simulink model "BugE_v0_40_MAS"  (R2015b)
settings: Solver=FixedStepDiscrete  StartTime=0.0  StopTime=inf  FixedStep=sample_time  RelTol=1e-3
values from neighbouring files (symbols this model uses):
  AB_diode_dV = 0.9    [main_sync.m]
  air_density = 1.225    [main_sync.m]
  bus_charger_Pmax = 1000    [main_sync.m]
  bus_load_Pmax_abs = 500    [main_sync.m]
  capInitVolt = capVmax*sqrt(capInitSoC)    [main_sync.m]
  cyc_kph = [cyc_kph(:,1), cyc_kph(:,2)*speed_max_limit/speed_max]    [main_sync.m]
  cyc_repeat = 0    [main_sync.m]
  ess1_init_soc = 1    [main_sync.m]
  ess1_soh = 1    [main_sync.m]
  ess2_init_soc = 1    [main_sync.m]
  ess2_soh = 1    [main_sync.m]
  ess3_init_soc = 1    [main_sync.m]
  ess3_soh = 1    [main_sync.m]
  ess4_init_soc = 1    [main_sync.m]
  ess4_soh = 1    [main_sync.m]
  ess5_init_soc = 1    [main_sync.m]
  ess5_soh = 1    [main_sync.m]
  gear_ratio = 6    [main_sync.m]
  loadpower = rawcsv(:,2)    [main_sync.m]
  loadtime = rawcsv(:,1)    [main_sync.m]
  lockSOCs = 0    [main_sync.m]
  max_brk_torque = 300    [main_sync.m]
  no_wheels = 3    [main_sync.m]
  period2 = max(loadtime)    [main_sync.m]
  PV_Pmax = 100    [main_sync.m]
  sample_time = 0.01    [main_sync.m]
  startup_seq_step_delay = 0.2    [main_sync.m]
  stop_option = 0    [main_sync.m]
  use_drive_cycle = 1    [main_sync.m]
  use_real_subs_loads = 1    [main_sync.m]
  vbus_max = 25    [main_sync.m]
  vbus_min = 17    [main_sync.m]
  vbus_safety_threshold = 2    [main_sync.m]
  vbus_threshold = 20    [main_sync.m]
  veh_CD = 0.35    [main_sync.m]
  veh_FA = 1.543    [main_sync.m]
  veh_gravity = 9.81*veh_mass    (= 1863.9)    [main_sync.m]
  veh_mass = 190    [main_sync.m]
  wh_1st_rrc = 0.02    [main_sync.m]
  wh_bearing_frc = 0.0015    [main_sync.m]
  wh_inertia = 0.0556    [main_sync.m]
  wh_radius = 0.508/2    (= 0.254)    [main_sync.m]
undefined symbols (not defined in the file or in its folder): capC, capR, cyc_acc, cyc_avg_time_samples, cyc_brk, cyc_grade, cyc_key, DCM_eff_factor_for_Vin, DCM_eff_for_Iout, DCM_Iout, DCM_Iout_max, DCM_Pin_noload, DCM_Pout_max, DCM_Vin, DCM_Vout, DiscIntNeverNeededParam, ess2_coulombic_eff, ess2_Ineg_max_SOC, ess2_Ineg_max_temp, ess2_Ipos_max_SOC, ess2_Ipos_max_temp, ess2_max_ah_cap, ess2_max_volts, ess2_min_volts, ess2_module_parallel, ess2_module_series, ess2_r_dis, ess2_soc, ess2_SOC_for_Ilimit, ess2_temp_for_Ilimit, ess2_temp_max, ess2_tmp, ess2_voc, ess3_coulombic_eff, ess3_max_ah_cap, ess3_module_parallel, ess3_module_series, ess3_r_dis, ess3_soc, ess3_tmp, ess3_voc, ess_coulombic_eff, ess_Ineg_max_SOC, ess_Ineg_max_temp, ess_Ipos_max_SOC, ess_Ipos_max_temp, ess_max_ah_cap, ess_max_volts, ess_min_volts, ess_module_parallel, ess_module_series, ess_nominal_volts, ess_r_dis, ess_soc, ess_SOC_for_Ilimit, ess_temp_for_Ilimit, ess_temp_max, ess_tmp, ess_voc, MC_eff1 ... (+17)
libraries: simulink x139, commfilt2 x1, simulink_extras x1
(part 6 of 7)

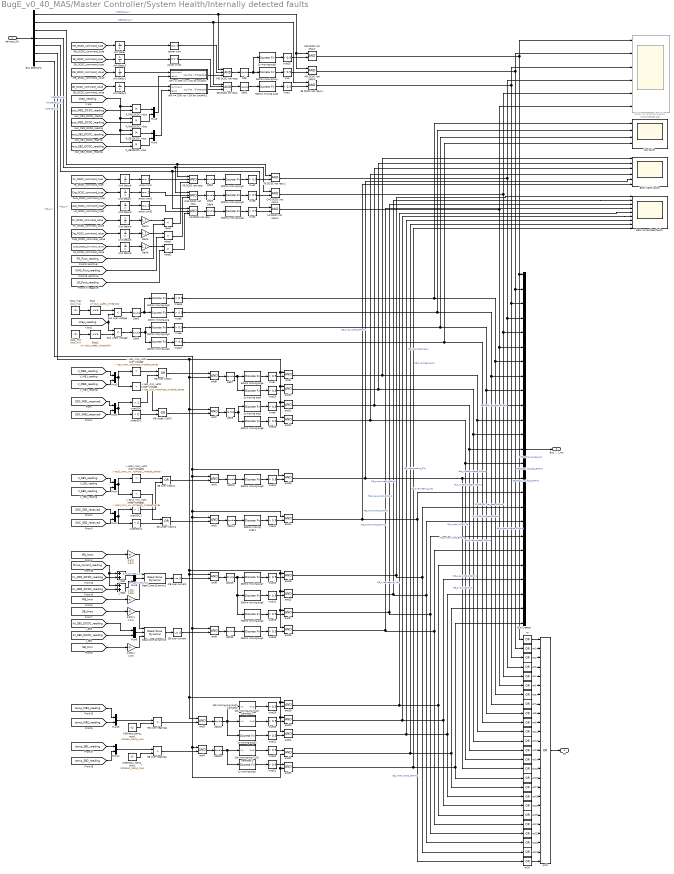
== system BugE_v0_40_MAS/Master Controller/System Health/Internally detected faults ==
  devices_ON : Inport
  0.90*ess2_temp_max1 : Constant  Value=0.9*ess2_temp_max  SampleTime=sample_time
  0.90*ess_temp_max1 : Constant  Value=0.9*ess_temp_max  SampleTime=sample_time
  "0.975 " : Gain  Gain=0.975
  0.975 1 : Gain  Gain=0.975
  "1.025 " : Gain  Gain=1.025
  1.025 1 : Gain  Gain=1.025
  1s moving avg{1..4,20} (5 alike) : DiscreteFir  Coefficients=ones(1,1*(1/sample_time))/(1*(1/sample_time))  SampleTime=sample_time
  200ms moving avg : DiscreteFir  Coefficients=ones(1,0.2*(1/sample_time))/(0.2*(1/sample_time))  SampleTime=sample_time
  200ms moving avg1 : DiscreteFir  Coefficients=ones(1,0.2*(1/sample_time))/(0.2*(1/sample_time))  SampleTime=sample_time
  20s moving avg (1/20 samples)1 : Subsystem
  20s moving avg (1/20 samples)3 : Subsystem
  250ms moving avg1 : DiscreteFir  Coefficients=ones(1,0.25*(1/sample_time))/(0.25*(1/sample_time))  SampleTime=sample_time
  250ms moving avg7 : DiscreteFir  Coefficients=ones(1,0.25*(1/sample_time))/(0.25*(1/sample_time))  SampleTime=sample_time
  2dbl{,1..7,9,12,14..16,19..20} (15 alike) : DataTypeConversion  OutDataTypeStr=double
  400ms moving avg1 : DiscreteFir  Coefficients=ones(1,0.4*(1/sample_time))/(0.4*(1/sample_time))  SampleTime=sample_time
  400ms moving avg2 : DiscreteFir  Coefficients=ones(1,0.4*(1/sample_time))/(0.4*(1/sample_time))  SampleTime=sample_time
  40s moving avg (1/40 samples) : Subsystem
  500ms moving avg{,1..6,8..9,11} (10 alike) : DiscreteFir  Coefficients=ones(1,0.5*(1/sample_time))/(0.5*(1/sample_time))  SampleTime=sample_time
  750ms moving avg2 : DiscreteFir  Coefficients=ones(1,0.75*(1/sample_time))/(0.75*(1/sample_time))  SampleTime=sample_time
  < ess2_min_volts under-voltage1 : simulink/Logic and Bit Operations/Compare To Constant  relop=<  const=ess2_min_volts*ess2_module_series  OutDataTypeStr=boolean
  < ess_min_volts under-voltage : simulink/Logic and Bit Operations/Compare To Constant  relop=<  const=ess_min_volts*ess_module_series  OutDataTypeStr=boolean
  > ess2_max_volts over-voltage1 : simulink/Logic and Bit Operations/Compare To Constant  relop=>  const=ess2_max_volts*ess2_module_series  OutDataTypeStr=boolean
  > ess_max_volts over-voltage : simulink/Logic and Bit Operations/Compare To Constant  relop=>  const=ess_max_volts*ess_module_series  OutDataTypeStr=boolean
  Batt V/SOC faults : Scope  NumInputPorts=6
  Batt current/heat faults : Scope  NumInputPorts=9
  Bias : Bias  Bias=vbus_safety_threshold
  Bias1 : Bias  Bias=-vbus_safety_threshold
  Bus Creator : BusCreator  Inputs=25
  Bus Selector3 : BusSelector  OutputSignals=MBDCDC_on,SBDCDC_on,FEDCDC_on,CHGDCDC_on,LDDCDC_on,MB_on,SB_on
  Bus over voltage : RelationalOperator  Operator=<  OutDataTypeStr=boolean
  Bus under voltage : RelationalOperator  Operator=<  OutDataTypeStr=boolean
  CHG DCDC not resp. : Logic  Inputs=3  AllPortsSameDT=off  OutDataTypeStr=boolean
  CHG DCDC not resp.1 : Logic  AllPortsSameDT=off  OutDataTypeStr=boolean
  DCDC not responding faults : Scope  Commented=on  NumInputPorts=6
  Dead Zone Dynamic2 : simulink/Discontinuities/Dead Zone Dynamic
  Dead Zone Dynamic3 : simulink/Discontinuities/Dead Zone Dynamic
  FE DCDC not resp. : Logic  Inputs=3  AllPortsSameDT=off  OutDataTypeStr=boolean
  FE DCDC not resp.1 : Logic  AllPortsSameDT=off  OutDataTypeStr=boolean
  Gain4 : Gain  Gain=1.1
  Gain5 : Gain  Gain=1.1
  Gain6 : Gain  Gain=1.1
  I_MB1 : Sum
  I_MB2 : Sum
  LD DCDC not resp. : Logic  Inputs=3  AllPortsSameDT=off  OutDataTypeStr=boolean
  LD DCDC not resp.1 : Logic  AllPortsSameDT=off  OutDataTypeStr=boolean
  MB over-heating1 : RelationalOperator  Operator=>  OutDataTypeStr=boolean
  MB DCDC not resp. : Logic  Inputs=3  AllPortsSameDT=off  OutDataTypeStr=boolean
  MB DCDC not resp.1 : Logic  AllPortsSameDT=off  OutDataTypeStr=boolean
  MB DCDC not resp.2 : Logic  AllPortsSameDT=off  OutDataTypeStr=boolean
  MB over V/SOC : Logic  Operator=OR  AllPortsSameDT=off  OutDataTypeStr=boolean
  MB over-current : simulink/Logic and Bit Operations/Compare To Zero  relop=~=  OutDataTypeStr=boolean
  MB under V/SOC : Logic  Operator=OR  AllPortsSameDT=off  OutDataTypeStr=boolean
  Mux{1..6,8..9,13..14} (10 alike) : Mux  Inputs=2
  P_MB1DCDC->bus : Product
  P_MB2DCDC->bus : Product
  P_SB1DCDC->bus : Product
  P_SB2DCDC->bus : Product
  SB over-heating1 : RelationalOperator  Operator=>  OutDataTypeStr=boolean
  SB DCDC not resp. : Logic  Inputs=3  AllPortsSameDT=off  OutDataTypeStr=boolean
  SB DCDC not resp.1 : Logic  AllPortsSameDT=off  OutDataTypeStr=boolean
  SB over V/SOC1 : Logic  Operator=OR  AllPortsSameDT=off  OutDataTypeStr=boolean
  SB over-current : simulink/Logic and Bit Operations/Compare To Zero  relop=~=  OutDataTypeStr=boolean
  SB under V/SOC1 : Logic  Operator=OR  AllPortsSameDT=off  OutDataTypeStr=boolean
  Unit Delay{,1..9} (10 alike) : UnitDelay  SampleTime=sample_time
  and{1..23} (23 alike) : Logic  AllPortsSameDT=off  OutDataTypeStr=boolean
  bus faults : Scope  NumInputPorts=4
  diff >= 10% (or >1W for cmd=0) : Subsystem
  diff >= 10% (or >1W for cmd=0)1 : Subsystem
  or{,1..9,11..25} (25 alike) : Logic  Operator=OR  Inputs=1  AllPortsSameDT=off  OutDataTypeStr=boolean
  or10 : Logic  Operator=OR  Inputs=25  AllPortsSameDT=off  OutDataTypeStr=boolean
  overSOC : simulink/Logic and Bit Operations/Compare To Constant  relop=>  const=1  OutDataTypeStr=boolean
  overSOC1 : simulink/Logic and Bit Operations/Compare To Constant  relop=>  const=1  OutDataTypeStr=boolean
  pmax cmd : simulink/Logic and Bit Operations/Compare To Constant  relop===  const=2  OutDataTypeStr=boolean
  pmax cmd1 : simulink/Logic and Bit Operations/Compare To Constant  relop===  const=2  OutDataTypeStr=boolean
  pmax cmd2 : simulink/Logic and Bit Operations/Compare To Constant  relop===  const=2  OutDataTypeStr=boolean
  power cmd : simulink/Logic and Bit Operations/Compare To Constant  relop===  const=0  OutDataTypeStr=boolean
  power cmd1 : simulink/Logic and Bit Operations/Compare To Constant  relop===  const=0  OutDataTypeStr=boolean
  relop : RelationalOperator  Operator=<  OutDataTypeStr=boolean
  relop1 : RelationalOperator  Operator=<  OutDataTypeStr=boolean
  relop2 : RelationalOperator  Operator=>  OutDataTypeStr=boolean
  true{,1..7,9..16,19..23,25..27,29} (25 alike) : simulink/Logic and Bit Operations/Compare To Constant  relop=>  const=0.5  OutDataTypeStr=boolean
  underSOC : simulink/Logic and Bit Operations/Compare To Constant  relop=<  const=0  OutDataTypeStr=boolean
  underSOC1 : simulink/Logic and Bit Operations/Compare To Constant  relop=<  const=0  OutDataTypeStr=boolean
  vbus_max : Constant  Value=vbus_max  SampleTime=sample_time
  vbus_min : Constant  Value=vbus_min  SampleTime=sample_time
  FD : Outport  SampleTime=sample_time
  Bus (...)_ms : Outport  Port=2  SampleTime=sample_time
  wires:
  diff >= 10% (or >1W for cmd=0)1/1(significant diff detected) -> SB DCDC not resp./3
  power cmd1/1 -> SB DCDC not resp./2
  Mux8/1 -> diff >= 10% (or >1W for cmd=0)/2(result)
  Mux9/1 -> diff >= 10% (or >1W for cmd=0)1/2(result)
  power cmd/1 -> MB DCDC not resp./2
  [MB_DCDC_command_type] -> Unit Delay/1
  [MB_DCDC_command_value] -> Unit Delay1/1
  [SB_DCDC_command_value] -> Unit Delay2/1
  [SB_DCDC_command_type] -> Unit Delay3/1
  [Iout_MB1_DCDC_reading] -> P_MB1DCDC->bus/2
  [Vcap_reading] -> P_MB1DCDC->bus/1, P_MB2DCDC->bus/1, P_SB1DCDC->bus/1, P_SB2DCDC->bus/1
  [Iout_MB2_DCDC_reading] -> P_MB2DCDC->bus/2
  [Iout_SB1_DCDC_reading] -> P_SB1DCDC->bus/2
  [Iout_SB2_DCDC_reading] -> P_SB2DCDC->bus/2
  Unit Delay/1 -> power cmd/1
  Unit Delay3/1 -> power cmd1/1
  P_MB1DCDC->bus/1 -> Mux8/1
  P_MB2DCDC->bus/1 -> Mux8/2
  P_SB1DCDC->bus/1 -> Mux9/1
  P_SB2DCDC->bus/1 -> Mux9/2
  Unit Delay1/1 -> diff >= 10% (or >1W for cmd=0)/1(command)
  Unit Delay2/1 -> diff >= 10% (or >1W for cmd=0)1/1(command)
  SB DCDC not resp./1 -> 2dbl1/1
  MB DCDC not resp./1 -> 2dbl/1
  vbus_min/1 -> Bias1/1
  vbus_max/1 -> Bias/1
  Bias/1 -> Bus over voltage/1
  [Vcap_reading] -> Bus over voltage/2, Bus under voltage/1
  Bias1/1 -> Bus under voltage/2
  [V_MB1_reading] -> Mux3/1
  [V_MB2_reading] -> Mux3/2
  [V_SB1_reading] -> Mux4/1
  [V_SB2_reading] -> Mux4/2
  [SOC_MB1_received] -> Mux1/1
  [SOC_MB2_received] -> Mux1/2
  Mux1/1 -> overSOC/1, underSOC/1
  Mux3/1 -> > ess_max_volts over-voltage/1, < ess_min_volts under-voltage/1
  > ess_max_volts over-voltage/1 -> MB over V/SOC/1
  overSOC/1 -> MB over V/SOC/2
  underSOC/1 -> MB under V/SOC/2
  < ess_min_volts under-voltage/1 -> MB under V/SOC/1
  [SOC_SB2_received] -> Mux2/2
  [SOC_SB1_received] -> Mux2/1
  and7/1 -> 2dbl9/1
  Mux5/1 -> Dead Zone Dynamic2/2
  [Iin_SB1_DCDC_reading] -> Mux6/1
  [Iin_SB2_DCDC_reading] -> Mux6/2
  Mux6/1 -> Dead Zone Dynamic3/2
  "0.975 "/1 -> Dead Zone Dynamic2/1
  "1.025 "/1 -> Dead Zone Dynamic2/3
  0.975 1/1 -> Dead Zone Dynamic3/1
  [MB_Imin] -> "1.025 "/1
  [MB_Imax] -> "0.975 "/1
  Dead Zone Dynamic3/1 -> SB over-current/1
  [Drive_current_reading] -> I_MB2/1, I_MB1/1
  [SB_Imax] -> 0.975 1/1
  [SB_Imin] -> 1.025 1/1
  1.025 1/1 -> Dead Zone Dynamic3/3
  I_MB1/1 -> Mux5/1  "ems_SH_MB1_Iout"
  [Iin_MB2_DCDC_reading] -> I_MB2/2
  [Iin_MB1_DCDC_reading] -> I_MB1/2
  I_MB2/1 -> Mux5/2  "ems_SH_MB2_Iout"
  [PV_DCDC_command_value] -> Unit Delay4/1
  [Chg_DCDC_command_value] -> Unit Delay5/1
  [PV_DCDC_command_type] -> Unit Delay6/1
  [Chg_DCDC_command_type] -> Unit Delay7/1
  [Load_DCDC_command_value] -> Unit Delay8/1
  [Load_DCDC_command_type] -> Unit Delay9/1
  Unit Delay6/1 -> pmax cmd/1
  Unit Delay7/1 -> pmax cmd1/1
  Unit Delay9/1 -> pmax cmd2/1
  Unit Delay4/1 -> Gain4/1
  Unit Delay5/1 -> Gain5/1
  Unit Delay8/1 -> Gain6/1
  Gain4/1 -> relop/1
  [FE_Pout_reading] -> relop/2
  Gain5/1 -> relop1/1
  [CHG_Pout_reading] -> relop1/2
  Gain6/1 -> relop2/1
  [LD_Pout_reading] -> relop2/2
  pmax cmd/1 -> FE DCDC not resp./2
  relop/1 -> FE DCDC not resp./3
  pmax cmd1/1 -> CHG DCDC not resp./2
  relop1/1 -> CHG DCDC not resp./3
  pmax cmd2/1 -> LD DCDC not resp./2
  relop2/1 -> LD DCDC not resp./3
  FE DCDC not resp./1 -> 2dbl2/1
  CHG DCDC not resp./1 -> 2dbl3/1
  LD DCDC not resp./1 -> 2dbl4/1
  500ms moving avg/1 -> true/1
  2dbl/1 -> 1s moving avg3/1, 500ms moving avg/1
  500ms moving avg1/1 -> true1/1
  2dbl1/1 -> 500ms moving avg1/1
  500ms moving avg2/1 -> true2/1
  2dbl2/1 -> 500ms moving avg2/1
  500ms moving avg3/1 -> true3/1
  2dbl3/1 -> 500ms moving avg3/1
  500ms moving avg4/1 -> true4/1
  2dbl4/1 -> 500ms moving avg4/1
  MB DCDC not resp.1/1 -> or1/1, Bus Creator/2, DCDC not responding faults/2  "MBDCDC_not_resp_500ms"
  FE DCDC not resp.1/1 -> or3/1, Bus Creator/4, DCDC not responding faults/4  "FEDCDC_not_resp_500ms"
  CHG DCDC not resp.1/1 -> or4/1, Bus Creator/5, DCDC not responding faults/5  "CHGDCDC_not_resp_500ms"
  LD DCDC not resp.1/1 -> or5/1, Bus Creator/6, DCDC not responding faults/6  "LD_DCDC_not_resp_500ms"
  200ms moving avg/1 -> true5/1
  2dbl5/1 -> 400ms moving avg2/1, 200ms moving avg/1
  true5/1 -> bus faults/2, or7/1, Bus Creator/8  "Bus_over-voltage_200ms"
  200ms moving avg1/1 -> true6/1
  2dbl6/1 -> 200ms moving avg1/1, 400ms moving avg1/1
  true6/1 -> bus faults/3, or8/1, Bus Creator/9  "Bus_under-voltage_200ms"
  500ms moving avg5/1 -> true7/1
  2dbl7/1 -> 1s moving avg4/1, 500ms moving avg5/1
  and5/1 -> Batt V/SOC faults/1, or11/1, Bus Creator/11  "MB_over_V/SOC_500ms"
  and10/1 -> Batt V/SOC faults/2, or12/1, Bus Creator/12  "MB_over_V/SOC_1s"
  1s moving avg2/1 -> true9/1
  and11/1 -> Batt V/SOC faults/3, or13/1, Bus Creator/13  "MB_under_V/SOC_1s"
  and12/1 -> Batt V/SOC faults/4, or14/1, Bus Creator/14  "MB_under_V/SOC_500ms"
  Mux2/1 -> overSOC1/1, underSOC1/1
  Mux4/1 -> > ess2_max_volts over-voltage1/1, < ess2_min_volts under-voltage1/1
  underSOC1/1 -> SB under V/SOC1/2
  < ess2_min_volts under-voltage1/1 -> SB under V/SOC1/1
  SB under V/SOC1/1 -> and2/2
  500ms moving avg9/1 -> true12/1
  2dbl12/1 -> 500ms moving avg9/1
  and13/1 -> Batt V/SOC faults/5, or15/1, Bus Creator/15  "SB_over_V/SOC_500ms"
  500ms moving avg11/1 -> true14/1
  2dbl14/1 -> 500ms moving avg11/1
  and14/1 -> Batt V/SOC faults/6, Bus Creator/16, or25/1  "SB_under_V/SOC_500ms"
  250ms moving avg7/1 -> true15/1
  2dbl15/1 -> 250ms moving avg7/1, 750ms moving avg2/1, 500ms moving avg6/1
  and8/1 -> 2dbl15/1
  and18/1 -> Batt current/heat faults/1, or24/1, Bus Creator/17  "MB_over-current_250ms"
  250ms moving avg1/1 -> true16/1
  2dbl16/1 -> 250ms moving avg1/1
  and9/1 -> 2dbl16/1
  and16/1 -> or21/1, Bus Creator/20, Batt current/heat faults/4  "SB_over-current_250ms"
  and21/1 -> or18/1, Bus Creator/23, Batt current/heat faults/7  "MB_over-heating_1s"
  and23/1 -> Batt current/heat faults/9, Bus Creator/25, or16/1  "SB_over-heating_1s"
  and20/1 -> or19/1, Bus Creator/22, Batt current/heat faults/6  "MB_over-heating_20s"
  and22/1 -> Batt current/heat faults/8, Bus Creator/24, or17/1  "SB_over-heating_20s"
  or10/1 -> FD/1
  or/1 -> or10/1
  or1/1 -> or10/2
  or2/1 -> or10/3
  or3/1 -> or10/4
  or4/1 -> or10/5
  or5/1 -> or10/6
  or6/1 -> or10/7
  or7/1 -> or10/8
  or8/1 -> or10/9
  or9/1 -> or10/10
  or11/1 -> or10/11
  or12/1 -> or10/12
  or13/1 -> or10/13
  or14/1 -> or10/14
  or15/1 -> or10/15
  or16/1 -> or10/16
  or17/1 -> or10/17
  or18/1 -> or10/18
  or19/1 -> or10/19
  or20/1 -> or10/20
  or21/1 -> or10/21
  true26/1 -> bus faults/1, or6/1, Bus Creator/7  "Bus_over-voltage_400ms"
  true27/1 -> bus faults/4, or9/1, Bus Creator/10  "Bus_under-voltage_400ms"
  Bus Creator/1 -> Bus (...)_ms/1
  1s moving avg4/1 -> true23/1
  500ms moving avg8/1 -> true10/1
  2dbl9/1 -> 1s moving avg2/1, 500ms moving avg8/1
  and15/1 -> Batt current/heat faults/2, or23/1, Bus Creator/18  "MB_over-current_500ms"
  500ms moving avg6/1 -> true11/1
  750ms moving avg2/1 -> true13/1
  and17/1 -> or22/1, Bus Creator/19, Batt current/heat faults/3  "MB_over-current_750ms"
  1s moving avg3/1 -> true25/1
  400ms moving avg2/1 -> true26/1
  400ms moving avg1/1 -> true27/1
  and19/1 -> Batt current/heat faults/5, or20/1, Bus Creator/21  "MB_over-heating_40s"
  or22/1 -> or10/22
  or23/1 -> or10/23
  or24/1 -> or10/24
  or25/1 -> or10/25
  > ess2_max_volts over-voltage1/1 -> SB over V/SOC1/1
  overSOC1/1 -> SB over V/SOC1/2
  diff >= 10% (or >1W for cmd=0)/1(significant diff detected) -> MB DCDC not resp./3
  Bus under voltage/1 -> 2dbl6/1
  Bus over voltage/1 -> 2dbl5/1
  SB over V/SOC1/1 -> and1/2
  devices_ON/1 -> Bus Selector3/1
  Bus Selector3/1 -> MB DCDC not resp.1/1, MB DCDC not resp.2/1, MB DCDC not resp./1  "<MBDCDC_on>"
  Bus Selector3/2 -> SB DCDC not resp.1/1, SB DCDC not resp./1  "<SBDCDC_on>"
  Bus Selector3/3 -> FE DCDC not resp.1/1, FE DCDC not resp./1  "<FEDCDC_on>"
  Bus Selector3/4 -> CHG DCDC not resp.1/1, CHG DCDC not resp./1  "<CHGDCDC_on>"
  Bus Selector3/5 -> LD DCDC not resp.1/1, LD DCDC not resp./1  "<LDDCDC_on>"
  Bus Selector3/6 -> and12/1, and11/1, and10/1, and5/1, and6/2, and7/1, and16/1, and17/1, and15/1, and18/1, and8/1, and21/1, and20/1, and19/1, and3/1  "<MB_on>"
  Bus Selector3/7 -> and13/1, and1/1, and14/1, and2/1, and22/2, and23/2, and4/1, and9/1  "<SB_on>"
  Mux13/1 -> MB over-heating1/1
  [temp_SB1_reading] -> Mux14/1
  Mux14/1 -> SB over-heating1/1
  [temp_MB1_reading] -> Mux13/1
  0.90*ess_temp_max1/1 -> MB over-heating1/2
  SB over-heating1/1 -> and4/2
  [temp_MB2_reading] -> Mux13/2
  0.90*ess2_temp_max1/1 -> SB over-heating1/2
  [temp_SB2_reading] -> Mux14/2
  MB over-heating1/1 -> and3/2
  1s moving avg20/1 -> true21/1
  2dbl19/1 -> 1s moving avg20/1, 20s moving avg (1/20 samples)1/1(In1), 40s moving avg (1/40 samples)/1(In1)
  1s moving avg1/1 -> true22/1
  2dbl20/1 -> 1s moving avg1/1, 20s moving avg (1/20 samples)3/1(In1)
  40s moving avg (1/40 samples)/1(Out1) -> true29/1
  20s moving avg (1/20 samples)1/1(Out1) -> true19/1
  20s moving avg (1/20 samples)3/1(Out1) -> true20/1
  MB DCDC not resp.2/1 -> DCDC not responding faults/1, or/1, Bus Creator/1  "MBDCDC_not_resp_1s"
  SB DCDC not resp.1/1 -> DCDC not responding faults/3, or2/1, Bus Creator/3  "SBDCDC_not_resp_500ms"
  and6/1 -> 2dbl7/1
  MB under V/SOC/1 -> and7/2
  and1/1 -> 2dbl12/1
  and2/1 -> 2dbl14/1
  MB over-current/1 -> and8/2
  SB over-current/1 -> and9/2
  and3/1 -> 2dbl19/1
  and4/1 -> 2dbl20/1
  true1/1 -> SB DCDC not resp.1/2
  true/1 -> MB DCDC not resp.1/2
  true25/1 -> MB DCDC not resp.2/2
  true2/1 -> FE DCDC not resp.1/2
  true3/1 -> CHG DCDC not resp.1/2
  true4/1 -> LD DCDC not resp.1/2
  true7/1 -> and5/2
  true23/1 -> and10/2
  true9/1 -> and11/2
  true10/1 -> and12/2
  true12/1 -> and13/2
  true14/1 -> and14/2
  true15/1 -> and18/2
  true11/1 -> and15/2
  true13/1 -> and17/2
  true16/1 -> and16/2
  true29/1 -> and19/2
  true19/1 -> and20/2
  true21/1 -> and21/2
  true20/1 -> and22/1
  true22/1 -> and23/1
  MB over V/SOC/1 -> and6/1
  Dead Zone Dynamic2/1 -> MB over-current/1

== system BugE_v0_40_MAS/Master Controller/System Health/MB current limits ==
  Imax : Product
  Imin : Product
  Mux3 : Mux  Inputs=2
  Mux5 : Mux  Inputs=2
  "SOC -> Imax" : Lookup_n-D  NumberOfTableDimensions=1  BreakpointsForDimension1=ess_SOC_for_Ilimit(:)  Table=ess_Ipos_max_SOC(:)*ess_module_parallel  ExtrapMethod=Clip  UseLastTableValue=on  InternalRulePriority=Speed  RndMeth=Simplest  InputSameDT=on
  "SOC -> Imin" : Lookup_n-D  NumberOfTableDimensions=1  BreakpointsForDimension1=ess_SOC_for_Ilimit(:)  Table=ess_Ineg_max_SOC(:)*ess_module_parallel  ExtrapMethod=Clip  UseLastTableValue=on  InternalRulePriority=Speed  RndMeth=Simplest  InputSameDT=on
  "Temp -> Imax factor" : Lookup_n-D  NumberOfTableDimensions=1  BreakpointsForDimension1=ess_temp_for_Ilimit(:)  Table=ess_Ipos_max_temp(:)/max(ess_Ipos_max_temp)  ExtrapMethod=Clip  UseLastTableValue=on  InternalRulePriority=Speed  RndMeth=Simplest  InputSameDT=on
  "Temp -> Imin (factor, 0-1)" : Lookup_n-D  NumberOfTableDimensions=1  BreakpointsForDimension1=ess_temp_for_Ilimit(:)  Table=ess_Ineg_max_temp(:)/min(ess_Ineg_max_temp)  ExtrapMethod=Clip  UseLastTableValue=on  InternalRulePriority=Speed  RndMeth=Simplest  InputSameDT=on
  I maximums : Outport
  I minimums : Outport  Port=2
  wires:
  Mux3/1 -> "SOC -> Imax"/1, "SOC -> Imin"/1
  "SOC -> Imax"/1 -> Imax/1
  Mux5/1 -> "Temp -> Imin (factor, 0-1)"/1, "Temp -> Imax factor"/1
  "Temp -> Imax factor"/1 -> Imax/2
  "SOC -> Imin"/1 -> Imin/1
  "Temp -> Imin (factor, 0-1)"/1 -> Imin/2
  Imax/1 -> I maximums/1
  Imin/1 -> I minimums/1
  [SOC_MB1_received] -> Mux3/1
  [SOC_MB2_received] -> Mux3/2
  [temp_MB2_reading] -> Mux5/2
  [temp_MB1_reading] -> Mux5/1

== system BugE_v0_40_MAS/Master Controller/System Health/SB current limits ==
  Imax : Product
  Imin : Product
  Mux6 : Mux  Inputs=2
  Mux7 : Mux  Inputs=2
  "SOC -> Imax" : Lookup_n-D  NumberOfTableDimensions=1  BreakpointsForDimension1=ess2_SOC_for_Ilimit(:)  Table=ess2_Ipos_max_SOC(:)*ess2_module_parallel  ExtrapMethod=Clip  UseLastTableValue=on  InternalRulePriority=Speed  RndMeth=Simplest  InputSameDT=on
  "SOC -> Imin" : Lookup_n-D  NumberOfTableDimensions=1  BreakpointsForDimension1=ess2_SOC_for_Ilimit(:)  Table=ess2_Ineg_max_SOC(:)*ess2_module_parallel  ExtrapMethod=Clip  UseLastTableValue=on  InternalRulePriority=Speed  RndMeth=Simplest  InputSameDT=on
  "Temp -> Imax" : Lookup_n-D  NumberOfTableDimensions=1  BreakpointsForDimension1=ess2_temp_for_Ilimit(:)  Table=ess2_Ipos_max_temp(:)/max(ess2_Ipos_max_temp)  ExtrapMethod=Clip  UseLastTableValue=on  InternalRulePriority=Speed  RndMeth=Simplest  InputSameDT=on
  "Temp -> Imin (factor, 0-1)" : Lookup_n-D  NumberOfTableDimensions=1  BreakpointsForDimension1=ess2_temp_for_Ilimit(:)  Table=ess2_Ineg_max_temp(:)/min(ess2_Ineg_max_temp)  ExtrapMethod=Clip  UseLastTableValue=on  InternalRulePriority=Speed  RndMeth=Simplest  InputSameDT=on
  I maximums : Outport
  I minimums : Outport  Port=2
  wires:
  Mux6/1 -> "SOC -> Imax"/1, "SOC -> Imin"/1
  "SOC -> Imax"/1 -> Imax/1
  Mux7/1 -> "Temp -> Imin (factor, 0-1)"/1, "Temp -> Imax"/1
  "Temp -> Imax"/1 -> Imax/2
  "SOC -> Imin"/1 -> Imin/1
  "Temp -> Imin (factor, 0-1)"/1 -> Imin/2
  Imax/1 -> I maximums/1
  Imin/1 -> I minimums/1
  [SOC_SB1_received] -> Mux6/1
  [SOC_SB2_received] -> Mux6/2
  [temp_SB2_reading] -> Mux7/2
  [temp_SB1_reading] -> Mux7/1

== system BugE_v0_40_MAS/Misc/Energy Calculations/Battery losses ==
  Add : Sum  Inputs=5
  Unit Delay : UnitDelay  SampleTime=-1
  Out1 : Outport
  wires:
  [E_batt_loss2] -> Add/2
  [E_batt_loss1] -> Add/1
  Add/1 -> Out1/1
  [E_batt_loss4] -> Add/4
  [E_batt_loss5] -> Unit Delay/1
  [E_batt_loss3] -> Add/3
  Unit Delay/1 -> Add/5

== system BugE_v0_40_MAS/Misc/Energy Calculations/Battery regen ==
  E_batt_regen : Sum  Inputs=5
  Scope : Scope  NumInputPorts=4
  Unit Delay : UnitDelay  SampleTime=-1
  Out1 : Outport
  wires:
  [E_batt_regen3] -> Scope/3, E_batt_regen/3
  [E_batt_regen4] -> Scope/4, E_batt_regen/4
  [E_batt_regen1] -> Scope/1, E_batt_regen/1
  E_batt_regen/1 -> Out1/1
  [E_batt_regen2] -> Scope/2, E_batt_regen/2
  [E_batt_regen5] -> Unit Delay/1
  Unit Delay/1 -> E_batt_regen/5

== system BugE_v0_40_MAS/Misc/Energy Calculations/DCDC losses ==
  Add4 : Sum  Inputs=5
  Unit Delay1 : UnitDelay  SampleTime=-1
  Out1 : Outport
  wires:
  [E_DAB3_loss] -> Add4/4
  [E_DAB4_loss] -> Add4/5
  Add4/1 -> Out1/1
  [E_DCM_loss] -> Unit Delay1/1
  [E_DAB2_loss] -> Add4/2
  [E_DAB1_loss] -> Add4/1
  Unit Delay1/1 -> Add4/3

== system BugE_v0_40_MAS/Misc/Energy Calculations/E_accessories ==
  Add : Sum
  Unit Delay : UnitDelay  SampleTime=-1
  Unit Delay1 : UnitDelay  SampleTime=-1
  Out1 : Outport
  wires:
  [E_accessories] -> Unit Delay/1
  Unit Delay/1 -> Add/1
  [E_ECU] -> Unit Delay1/1
  Unit Delay1/1 -> Add/2
  Add/1 -> Out1/1

== system BugE_v0_40_MAS/Misc/Energy Calculations/E_battery_total ==
  Battery losses : Subsystem
  Battery useful : Subsystem
  E_battery_total : Sum
  Out1 : Outport
  wires:
  Battery losses/1(Out1) -> E_battery_total/2
  E_battery_total/1 -> Out1/1
  Battery useful/1(Out1) -> E_battery_total/1

== system BugE_v0_40_MAS/Misc/Energy Calculations/E_cap_total ==
  E_cap_total : Sum
  Out1 : Outport
  wires:
  [E_cap_useful] -> E_cap_total/2
  E_cap_total/1 -> Out1/1
  [E_cap_loss] -> E_cap_total/1

== system BugE_v0_40_MAS/Misc/Energy Calculations/E_vehicle_drive ==
  E_drive : Sum  Inputs=2
  Out1 : Outport
  wires:
  [E_acceleration] -> E_drive/1
  [E_climb] -> E_drive/2
  E_drive/1 -> Out1/1

== system BugE_v0_40_MAS/Misc/Energy Calculations/E_vehicle_friction ==
  E_friction : Sum  Inputs=2
  Out1 : Outport
  wires:
  [E_aero] -> E_friction/1
  [E_roll] -> E_friction/2
  E_friction/1 -> Out1/1

== system BugE_v0_40_MAS/Misc/Energy Calculations/Powertrain mech. losses ==
  E_friction1 : Sum  Inputs=3
  Mux : Mux  Inputs=3
  energy balance : Scope
  Out1 : Outport
  wires:
  [E_wh_bearing] -> E_friction1/3, Mux/3
  [E_motor_inertia] -> Mux/2, E_friction1/2
  [E_wh_inertia] -> Mux/1, E_friction1/1
  E_friction1/1 -> Out1/1
  Mux/1 -> energy balance/1

== system BugE_v0_40_MAS/Vehicle/Achievable vehicle speed/Energy Quantification1 ==
  Froll : Inport
  Fclimb : Inport  Port=2
  Ftract : Inport  Port=3
  Vi : Inport  Port=4
  > 0 : Saturate  UpperLimit=inf  LowerLimit=0
  "> 0 " : Saturate  UpperLimit=inf  LowerLimit=0
  acceleration : Sum  Inputs=---+
  aero : Product  Inputs=4  SaturateOnIntegerOverflow=on  RndMeth=Zero  InputSameDT=on  OutDataTypeStr=Inherit: Same as first input
  aero3 : Constant  Value=0.5*air_density*veh_CD*veh_FA  SampleTime=sample_time
  climb : Product  Inputs=**  SaturateOnIntegerOverflow=on  RndMeth=Zero  InputSameDT=on  OutDataTypeStr=Inherit: Same as first input
  power : Product  Inputs=**
  roll : Product  Inputs=**  SaturateOnIntegerOverflow=on  RndMeth=Zero  InputSameDT=on  OutDataTypeStr=Inherit: Same as first input
  tag scope: E_acceleration=global, E_aero=global, E_climb=global, E_roll=global
  wires:
  aero/1 -> acceleration/1, [E_aero]
  roll/1 -> acceleration/2, [E_roll]
  climb/1 -> acceleration/3, [E_climb]
  > 0/1 -> climb/2
  power/1 -> acceleration/4
  acceleration/1 -> "> 0 "/1
  "> 0 "/1 -> [E_acceleration]
  aero3/1 -> aero/1
  Vi/1 -> roll/1, power/1, climb/1, aero/2, aero/3, aero/4
  Froll/1 -> roll/2
  Fclimb/1 -> > 0/1
  Ftract/1 -> power/2

== system BugE_v0_40_MAS/Auxiliaries (LV Grid)/AB (w// diode)/Calculate SOC/Resettable Integrator ==
  input : Inport
  IC : Inport  Port=2
  Logical Operator : Logic  Operator=NOT  AllPortsSameDT=off  OutDataTypeStr=boolean
  Merge : Merge
  Subsystem : Subsystem
  Subsystem1 : Subsystem
  Unit Delay : UnitDelay  SampleTime=-1
  nochange : RelationalOperator  Operator===  OutDataTypeStr=boolean
  Out1 : Outport
  wires:
  IC/1 -> nochange/2, Unit Delay/1, Subsystem/2(IC)
  Merge/1 -> Out1/1
  Subsystem1/1(Out1) -> Merge/2
  Subsystem/1(Out1) -> Merge/1
  input/1 -> Subsystem/1(input)
  nochange/1 -> Subsystem/Enable, Logical Operator/1
  Unit Delay/1 -> nochange/1
  Logical Operator/1 -> Subsystem1/Enable

== system BugE_v0_40_MAS/Energy Storage (New Grid)/MB1/Calculate SOC/Resettable Integrator ==
  input : Inport
  IC : Inport  Port=2
  Logical Operator : Logic  Operator=NOT  AllPortsSameDT=off  OutDataTypeStr=boolean
  Merge : Merge
  Subsystem : Subsystem
  Subsystem1 : Subsystem
  Unit Delay : UnitDelay  SampleTime=-1
  nochange : RelationalOperator  Operator===  OutDataTypeStr=boolean
  Out1 : Outport
  wires:
  IC/1 -> nochange/2, Unit Delay/1, Subsystem/2(IC)
  Merge/1 -> Out1/1
  Subsystem1/1(Out1) -> Merge/2
  Subsystem/1(Out1) -> Merge/1
  input/1 -> Subsystem/1(input)
  nochange/1 -> Subsystem/Enable, Logical Operator/1
  Unit Delay/1 -> nochange/1
  Logical Operator/1 -> Subsystem1/Enable

== system BugE_v0_40_MAS/Energy Storage (New Grid)/MB2/Calculate SOC/Resettable Integrator ==
  input : Inport
  IC : Inport  Port=2
  Logical Operator : Logic  Operator=NOT  AllPortsSameDT=off  OutDataTypeStr=boolean
  Merge : Merge
  Subsystem : Subsystem
  Subsystem1 : Subsystem
  Unit Delay : UnitDelay  SampleTime=-1
  nochange : RelationalOperator  Operator===  OutDataTypeStr=boolean
  Out1 : Outport
  wires:
  IC/1 -> nochange/2, Unit Delay/1, Subsystem/2(IC)
  Merge/1 -> Out1/1
  Subsystem1/1(Out1) -> Merge/2
  Subsystem/1(Out1) -> Merge/1
  input/1 -> Subsystem/1(input)
  nochange/1 -> Subsystem/Enable, Logical Operator/1
  Unit Delay/1 -> nochange/1
  Logical Operator/1 -> Subsystem1/Enable

== system BugE_v0_40_MAS/Inputs Hardware to Controller/User Inputs/Command Cycles (no regenerative braking assumed)/drive_cycle ==
  time : Inport
  repeat : Inport  Port=2
  velocity kph : Inport  Port=3
  Add : Sum  Inputs=+-
  Delay : Delay  DelayLength=cyc_avg_time_samples  SampleTime=sample_time
  Discrete PID : simulink/Continuous/PID Controller  Controller=PI  TimeDomain=Discrete-time  SampleTime=sample_time  IntegratorMethod=Forward Euler  FilterMethod=Forward Euler  Form=Parallel  UseFilter=on  ControllerParametersSource=internal  P=0.4  I=0.04  D=0  N=100  InitialConditionSource=internal  InitialConditionForIntegrator=0  InitialConditionForFilter=0  ExternalReset=none  LimitOutput=on  UpperSaturationLimit=1  LowerSaturationLimit=-1  LinearizeAsGain=off  AntiWindupMode=back-calculation  Kb=1  TrackingMode=off  Kt=1  PParamMin=[]  PParamMax=[]  IParamMin=[]  IParamMax=[]  DParamMin=[]  DParamMax=[]  NParamMin=[]  NParamMax=[]  KbParamMin=[]  KbParamMax=[]  KtParamMin=[]  KtParamMax=[]  POutMin=[]  POutMax=[]  IOutMin=[]  IOutMax=[]  DOutMin=[]  DOutMax=[]  NOutMin=[]  NOutMax=[]  KbOutMin=[]  KbOutMax=[]  KtOutMin=[]  KtOutMax=[]  IntegratorOutMin=[]  IntegratorOutMax=[]  FilterOutMin=[]  FilterOutMax=[]  SumOutMin=[]  SumOutMax=[]  SumI1OutMin=[]  SumI1OutMax=[]  SumI2OutMin=[]  SumI2OutMax=[]  SumI3OutMin=[]  SumI3OutMax=[]  SumDOutMin=[]  SumDOutMax=[]  SaturationOutMin=[]  SaturationOutMax=[]  IntegratorContinuousStateAttributes=''  IntegratorStateMustResolveToSignalObject=off  IntegratorRTWStateStorageClass=Auto  FilterContinuousStateAttributes=''  FilterStateMustResolveToSignalObject=off  FilterRTWStateStorageClass=Auto  DifferentiatorICPrevScaledInput=0  DifferentiatorOutMin=[]  DifferentiatorOutMax=[]
  Discrete-Time Integrator1 : DiscreteIntegrator  InitialConditionSetting=State (most efficient)  SampleTime=sample_time  ICPrevOutput=DiscIntNeverNeededParam  ICPrevScaledInput=DiscIntNeverNeededParam
  From Workspace4 : FromWorkspace  VariableName=cyc_kph_ts  SampleTime=sample_time
  Gain : Gain  Gain=-1
  Look-Up Table4 : Lookup_n-D  NumberOfTableDimensions=1  BreakpointsForDimension1=cyc_kph(:,1)  Table=cyc_kph(:,2)  InternalRulePriority=Speed  SaturateOnIntegerOverflow=on  InputSameDT=on
  Mux1 : Mux  Inputs=2
  Mux2 : Mux  Inputs=2
  Unit Delay : UnitDelay  SampleTime=-1
  V diff : Sum  Inputs=+-
  Velocity Tracing : Scope
  acc : Saturate  UpperLimit=1  LowerLimit=0
  brk : Saturate  UpperLimit=0  LowerLimit=-1
  cyc_avg_time_samples : Constant  Value=cyc_avg_time_samples*sample_time  SampleTime=sample_time
  vel km/h : Switch  Criteria=u2 > Threshold
  velocity command : Product  Inputs=/*
  acc/brk : Outport
  wires:
  From Workspace4/1 -> vel km/h/3
  Look-Up Table4/1 -> vel km/h/1
  cyc_avg_time_samples/1 -> velocity command/1
  velocity command/1 -> Mux1/1, V diff/1
  vel km/h/1 -> Discrete-Time Integrator1/1
  repeat/1 -> vel km/h/2
  time/1 -> Look-Up Table4/1
  V diff/1 -> Discrete PID/1
  Discrete PID/1 -> acc/1, brk/1
  acc/1 -> Mux2/1
  brk/1 -> Gain/1
  velocity kph/1 -> Unit Delay/1
  Gain/1 -> Mux2/2
  Unit Delay/1 -> Mux1/2, V diff/2
  Discrete-Time Integrator1/1 -> Delay/1, Add/1
  Delay/1 -> Add/2
  Add/1 -> velocity command/2
  Mux1/1 -> Velocity Tracing/1
  Mux2/1 -> acc/brk/1

== system BugE_v0_40_MAS/Inputs Hardware to Controller/User Inputs/Command Cycles (no regenerative braking assumed)/key ==
  time : Inport
  repeat : Inport  Port=2
  Constant2 : Constant  Value=2  SampleTime=sample_time
  From Workspace3 : FromWorkspace  VariableName=cyc_key_ts  SampleTime=sample_time  Interpolate=off  OutputAfterFinalValue=Holding final value
  Look-Up Table3 : Lookup_n-D  NumberOfTableDimensions=1  BreakpointsForDimension1=cyc_key(:,1)  Table=cyc_key(:,2)  InterpMethod=Flat  InternalRulePriority=Speed  SaturateOnIntegerOverflow=on  InputSameDT=on
  "key " : Switch  Criteria=u2 > Threshold
  motor on : RelationalOperator  Operator===  OutDataTypeStr=boolean
  key : Outport
  motor_on : Outport  Port=2
  wires:
  Look-Up Table3/1 -> "key "/1
  From Workspace3/1 -> "key "/3
  "key "/1 -> key/1, motor on/1
  Constant2/1 -> motor on/2
  motor on/1 -> motor_on/1
  time/1 -> Look-Up Table3/1
  repeat/1 -> "key "/2

== system BugE_v0_40_MAS/Inputs Hardware to Controller/User Inputs/Command Cycles (no regenerative braking assumed)/pedal cycle ==
  motor_on : Inport
  time : Inport  Port=2
  repeat : Inport  Port=3
  "  1/100" : Gain  Gain=1/100
  1/100 : Gain  Gain=1/100
  Add : Sum  Inputs=+-
  Add1 : Sum  Inputs=+-
  Constant4 : Constant  Value=0  SampleTime=sample_time
  Delay : Delay  DelayLength=cyc_avg_time_samples  SampleTime=sample_time
  Delay1 : Delay  DelayLength=cyc_avg_time_samples  SampleTime=sample_time
  Discrete-Time Integrator : DiscreteIntegrator  InitialConditionSetting=State (most efficient)  SampleTime=sample_time  ICPrevOutput=DiscIntNeverNeededParam  ICPrevScaledInput=DiscIntNeverNeededParam
  Discrete-Time Integrator1 : DiscreteIntegrator  InitialConditionSetting=State (most efficient)  SampleTime=sample_time  ICPrevOutput=DiscIntNeverNeededParam  ICPrevScaledInput=DiscIntNeverNeededParam
  From Workspace : FromWorkspace  VariableName=cyc_acc_ts  SampleTime=sample_time
  From Workspace2 : FromWorkspace  VariableName=cyc_brk_ts  SampleTime=sample_time
  Look-Up Table : Lookup_n-D  NumberOfTableDimensions=1  BreakpointsForDimension1=cyc_acc(:,1)  Table=cyc_acc(:,2)  InternalRulePriority=Speed  SaturateOnIntegerOverflow=on  InputSameDT=on
  Look-Up Table2 : Lookup_n-D  NumberOfTableDimensions=1  BreakpointsForDimension1=cyc_brk(:,1)  Table=cyc_brk(:,2)  InternalRulePriority=Speed  SaturateOnIntegerOverflow=on  InputSameDT=on
  Mux2 : Mux  Inputs=2
  Switch : Switch  Criteria=u2 > Threshold
  Switch3 : Switch  Criteria=u2 > Threshold
  acceleration : Switch  Criteria=u2 > Threshold
  brake : Switch  Criteria=u2 > Threshold
  cyc_avg_time_samples : Constant  Value=cyc_avg_time_samples*sample_time  SampleTime=sample_time
  moving avg acc % : Product  Inputs=/*
  moving avg brk % : Product  Inputs=*/
  acc/brk : Outport
  wires:
  Discrete-Time Integrator1/1 -> Delay1/1, Add/1
  Delay1/1 -> Add/2
  Add/1 -> moving avg acc %/2
  cyc_avg_time_samples/1 -> moving avg acc %/1, moving avg brk %/2
  Look-Up Table/1 -> Switch/1
  From Workspace/1 -> Switch/3
  Discrete-Time Integrator/1 -> Delay/1, Add1/1
  Delay/1 -> Add1/2
  Add1/1 -> moving avg brk %/1
  Look-Up Table2/1 -> Switch3/1
  From Workspace2/1 -> Switch3/3
  "  1/100"/1 -> Discrete-Time Integrator/1
  Switch3/1 -> "  1/100"/1
  1/100/1 -> Discrete-Time Integrator1/1
  Switch/1 -> 1/100/1
  moving avg brk %/1 -> brake/1
  moving avg acc %/1 -> acceleration/1
  Constant4/1 -> acceleration/3, brake/3
  motor_on/1 -> acceleration/2, brake/2
  time/1 -> Look-Up Table/1, Look-Up Table2/1
  repeat/1 -> Switch/2, Switch3/2
  acceleration/1 -> Mux2/1
  Mux2/1 -> acc/brk/1
  brake/1 -> Mux2/2

== system BugE_v0_40_MAS/Master Controller/Operating Mode Controller/Accessories (State 2)/pass ==
  I : Inport
  Logical Operator : Logic  Operator=NOT  AllPortsSameDT=off  OutDataTypeStr=boolean
  Logical Operator1 : Logic  Operator=NOT  AllPortsSameDT=off  OutDataTypeStr=boolean
  O : Outport
  wires:
  I/1 -> Logical Operator/1
  Logical Operator1/1 -> O/1
  Logical Operator/1 -> Logical Operator1/1

== system BugE_v0_40_MAS/Master Controller/Operating Mode Controller/Accessories (State 2)/pass5 ==
  I : Inport
  Logical Operator : Logic  Operator=NOT  AllPortsSameDT=off  OutDataTypeStr=boolean
  Logical Operator1 : Logic  Operator=NOT  AllPortsSameDT=off  OutDataTypeStr=boolean
  O : Outport
  wires:
  I/1 -> Logical Operator/1
  Logical Operator1/1 -> O/1
  Logical Operator/1 -> Logical Operator1/1

== system BugE_v0_40_MAS/Master Controller/Operating Mode Controller/Accessories (State 2)/pass6 ==
  I : Inport
  Logical Operator : Logic  Operator=NOT  AllPortsSameDT=off  OutDataTypeStr=boolean
  Logical Operator1 : Logic  Operator=NOT  AllPortsSameDT=off  OutDataTypeStr=boolean
  O : Outport
  wires:
  I/1 -> Logical Operator/1
  Logical Operator1/1 -> O/1
  Logical Operator/1 -> Logical Operator1/1

== system BugE_v0_40_MAS/Master Controller/Operating Mode Controller/Accessories (State 2)/pass7 ==
  I : Inport
  Logical Operator : Logic  Operator=NOT  AllPortsSameDT=off  OutDataTypeStr=boolean
  Logical Operator1 : Logic  Operator=NOT  AllPortsSameDT=off  OutDataTypeStr=boolean
  O : Outport
  wires:
  I/1 -> Logical Operator/1
  Logical Operator1/1 -> O/1
  Logical Operator/1 -> Logical Operator1/1

== system BugE_v0_40_MAS/Master Controller/Operating Mode Controller/Standby (State 0)/ones ==
  I : Inport
  Bias2 : Bias  Bias=1
  Gain2 : Gain  Gain=0
  bool2dbl2 : DataTypeConversion  OutDataTypeStr=double
  dbl2bool2 : DataTypeConversion  OutDataTypeStr=boolean
  O : Outport
  wires:
  bool2dbl2/1 -> Gain2/1
  Gain2/1 -> Bias2/1
  Bias2/1 -> dbl2bool2/1
  I/1 -> bool2dbl2/1
  dbl2bool2/1 -> O/1

== system BugE_v0_40_MAS/Master Controller/Operating Mode Controller/Standby (State 0)/ones1 ==
  I : Inport
  Bias2 : Bias  Bias=1
  Gain2 : Gain  Gain=0
  bool2dbl2 : DataTypeConversion  OutDataTypeStr=double
  dbl2bool2 : DataTypeConversion  OutDataTypeStr=boolean
  O : Outport
  wires:
  bool2dbl2/1 -> Gain2/1
  Gain2/1 -> Bias2/1
  Bias2/1 -> dbl2bool2/1
  I/1 -> bool2dbl2/1
  dbl2bool2/1 -> O/1

== system BugE_v0_40_MAS/Master Controller/Operating Mode Controller/Standby (State 0)/ones2 ==
  I : Inport
  Bias2 : Bias  Bias=1
  Gain2 : Gain  Gain=0
  bool2dbl2 : DataTypeConversion  OutDataTypeStr=double
  dbl2bool2 : DataTypeConversion  OutDataTypeStr=boolean
  O : Outport
  wires:
  bool2dbl2/1 -> Gain2/1
  Gain2/1 -> Bias2/1
  Bias2/1 -> dbl2bool2/1
  I/1 -> bool2dbl2/1
  dbl2bool2/1 -> O/1

== system BugE_v0_40_MAS/Master Controller/Operating Mode Controller/Standby (State 0)/ones3 ==
  I : Inport
  Bias2 : Bias  Bias=1
  Gain2 : Gain  Gain=0
  bool2dbl2 : DataTypeConversion  OutDataTypeStr=double
  dbl2bool2 : DataTypeConversion  OutDataTypeStr=boolean
  O : Outport
  wires:
  bool2dbl2/1 -> Gain2/1
  Gain2/1 -> Bias2/1
  Bias2/1 -> dbl2bool2/1
  I/1 -> bool2dbl2/1
  dbl2bool2/1 -> O/1

== system BugE_v0_40_MAS/Master Controller/Operating Mode Controller/Standby (State 0)/ones4 ==
  I : Inport
  Bias2 : Bias  Bias=1
  Gain2 : Gain  Gain=0
  bool2dbl2 : DataTypeConversion  OutDataTypeStr=double
  dbl2bool2 : DataTypeConversion  OutDataTypeStr=boolean
  O : Outport
  wires:
  bool2dbl2/1 -> Gain2/1
  Gain2/1 -> Bias2/1
  Bias2/1 -> dbl2bool2/1
  I/1 -> bool2dbl2/1
  dbl2bool2/1 -> O/1

== system BugE_v0_40_MAS/Master Controller/Operating Mode Controller/Startup sequence (State 1)/choose_droop_activations ==
  note: No loads or MB modules
      | where the DCDC is ok but
      | the battery is not usable
  devices_ON bus : Inport
  Enable : EnablePort  StatesWhenEnabling=reset
  Bus Creator : BusCreator  Inputs=5
  Bus Selector : BusSelector  OutputSignals=MBDCDC_on,MB_on,SBDCDC_on,SB_on,FEDCDC_on,FE_on,CHGDCDC_on,CHG_on,LDDCDC_on,LD_on
  Gain2 : Gain  Gain=0
  and{,1..4} (5 alike) : Logic  AllPortsSameDT=off  OutDataTypeStr=boolean
  bool2dbl2 : DataTypeConversion  OutDataTypeStr=double
  dbl2bool2 : DataTypeConversion  OutDataTypeStr=boolean
  droop_EN bus : Outport
  wires:
  devices_ON bus/1 -> Bus Selector/1
  and/1 -> Bus Creator/1  "MB_droop_EN"
  and2/1 -> Bus Creator/3  "FE_droop_EN"
  and3/1 -> Bus Creator/4  "CHG_droop_EN"
  and1/1 -> Bus Creator/2  "SB_droop_EN"
  Bus Creator/1 -> droop_EN bus/1
  dbl2bool2/1 -> Bus Creator/5  "LD_droop_EN"
  Bus Selector/1 -> and/1  "<MBDCDC_on>"
  Bus Selector/10 -> and4/2  "<LD_on>"
  Bus Selector/9 -> and4/1  "<LDDCDC_on>"
  Bus Selector/8 -> and3/2  "<CHG_on>"
  Bus Selector/7 -> and3/1  "<CHGDCDC_on>"
  Bus Selector/6 -> and2/2  "<FE_on>"
  Bus Selector/5 -> and2/1  "<FEDCDC_on>"
  Bus Selector/4 -> and1/2  "<SB_on>"
  Bus Selector/3 -> and1/1  "<SBDCDC_on>"
  Bus Selector/2 -> and/2  "<MB_on>"
  bool2dbl2/1 -> Gain2/1
  Gain2/1 -> dbl2bool2/1
  and4/1 -> bool2dbl2/1

== system BugE_v0_40_MAS/Master Controller/Operating Mode Controller/Startup sequence (State 1)/choose_droop_activations1 ==
  note: No MB modules where
      | the DCDC is ok but
      | the battery is not usable
  devices_ON bus : Inport
  Enable : EnablePort  StatesWhenEnabling=reset
  Bus Creator : BusCreator  Inputs=5
  Bus Selector : BusSelector  OutputSignals=MBDCDC_on,MB_on,SBDCDC_on,SB_on,FEDCDC_on,FE_on,CHGDCDC_on,CHG_on,LDDCDC_on,LD_on
  and{,1..4} (5 alike) : Logic  AllPortsSameDT=off  OutDataTypeStr=boolean
  droop_EN bus : Outport
  wires:
  devices_ON bus/1 -> Bus Selector/1
  and/1 -> Bus Creator/1  "MB_droop_EN"
  and2/1 -> Bus Creator/3  "FE_droop_EN"
  and3/1 -> Bus Creator/4  "CHG_droop_EN"
  and1/1 -> Bus Creator/2  "SB_droop_EN"
  Bus Creator/1 -> droop_EN bus/1
  and4/1 -> Bus Creator/5  "LD_droop_EN"
  Bus Selector/1 -> and/1  "<MBDCDC_on>"
  Bus Selector/10 -> and4/2  "<LD_on>"
  Bus Selector/9 -> and4/1  "<LDDCDC_on>"
  Bus Selector/8 -> and3/2  "<CHG_on>"
  Bus Selector/7 -> and3/1  "<CHGDCDC_on>"
  Bus Selector/6 -> and2/2  "<FE_on>"
  Bus Selector/5 -> and2/1  "<FEDCDC_on>"
  Bus Selector/4 -> and1/2  "<SB_on>"
  Bus Selector/3 -> and1/1  "<SBDCDC_on>"
  Bus Selector/2 -> and/2  "<MB_on>"

== system BugE_v0_40_MAS/Master Controller/Operating Mode Controller/Startup sequence (State 1)/ones ==
  I : Inport
  Bias2 : Bias  Bias=1
  Gain2 : Gain  Gain=0
  bool2dbl2 : DataTypeConversion  OutDataTypeStr=double
  dbl2bool2 : DataTypeConversion  OutDataTypeStr=boolean
  O : Outport
  wires:
  bool2dbl2/1 -> Gain2/1
  Gain2/1 -> Bias2/1
  Bias2/1 -> dbl2bool2/1
  I/1 -> bool2dbl2/1
  dbl2bool2/1 -> O/1

== system BugE_v0_40_MAS/Master Controller/Operating Mode Controller/Startup sequence (State 1)/ones1 ==
  I : Inport
  Bias2 : Bias  Bias=1
  Gain2 : Gain  Gain=0
  bool2dbl2 : DataTypeConversion  OutDataTypeStr=double
  dbl2bool2 : DataTypeConversion  OutDataTypeStr=boolean
  O : Outport
  wires:
  bool2dbl2/1 -> Gain2/1
  Gain2/1 -> Bias2/1
  Bias2/1 -> dbl2bool2/1
  I/1 -> bool2dbl2/1
  dbl2bool2/1 -> O/1

== system BugE_v0_40_MAS/Master Controller/Operating Mode Controller/Startup sequence (State 1)/ones2 ==
  I : Inport
  Bias2 : Bias  Bias=1
  Gain2 : Gain  Gain=0
  bool2dbl2 : DataTypeConversion  OutDataTypeStr=double
  dbl2bool2 : DataTypeConversion  OutDataTypeStr=boolean
  O : Outport
  wires:
  bool2dbl2/1 -> Gain2/1
  Gain2/1 -> Bias2/1
  Bias2/1 -> dbl2bool2/1
  I/1 -> bool2dbl2/1
  dbl2bool2/1 -> O/1

== system BugE_v0_40_MAS/Master Controller/Operating Mode Controller/Startup sequence (State 1)/ones3 ==
  I : Inport
  Bias2 : Bias  Bias=1
  Gain2 : Gain  Gain=0
  bool2dbl2 : DataTypeConversion  OutDataTypeStr=double
  dbl2bool2 : DataTypeConversion  OutDataTypeStr=boolean
  O : Outport
  wires:
  bool2dbl2/1 -> Gain2/1
  Gain2/1 -> Bias2/1
  Bias2/1 -> dbl2bool2/1
  I/1 -> bool2dbl2/1
  dbl2bool2/1 -> O/1

== system BugE_v0_40_MAS/Master Controller/Operating Mode Controller/Startup sequence (State 1)/ones4 ==
  I : Inport
  Bias2 : Bias  Bias=1
  Gain2 : Gain  Gain=0
  bool2dbl2 : DataTypeConversion  OutDataTypeStr=double
  dbl2bool2 : DataTypeConversion  OutDataTypeStr=boolean
  O : Outport
  wires:
  bool2dbl2/1 -> Gain2/1
  Gain2/1 -> Bias2/1
  Bias2/1 -> dbl2bool2/1
  I/1 -> bool2dbl2/1
  dbl2bool2/1 -> O/1

== system BugE_v0_40_MAS/Master Controller/Operating Mode Controller/Startup sequence (State 1)/pass ==
  I : Inport
  Logical Operator : Logic  Operator=NOT  AllPortsSameDT=off  OutDataTypeStr=boolean
  Logical Operator1 : Logic  Operator=NOT  AllPortsSameDT=off  OutDataTypeStr=boolean
  O : Outport
  wires:
  I/1 -> Logical Operator/1
  Logical Operator1/1 -> O/1
  Logical Operator/1 -> Logical Operator1/1

== system BugE_v0_40_MAS/Master Controller/Operating Mode Controller/Startup sequence (State 1)/pass1 ==
  I : Inport
  Logical Operator : Logic  Operator=NOT  AllPortsSameDT=off  OutDataTypeStr=boolean
  Logical Operator1 : Logic  Operator=NOT  AllPortsSameDT=off  OutDataTypeStr=boolean
  O : Outport
  wires:
  I/1 -> Logical Operator/1
  Logical Operator1/1 -> O/1
  Logical Operator/1 -> Logical Operator1/1

== system BugE_v0_40_MAS/Master Controller/Operating Mode Controller/Startup sequence (State 1)/startup_seq_step_delay w// latch ==
  sigin : Inport
  bus ready : Inport  Port=2
  2dbl : DataTypeConversion  OutDataTypeStr=double
  2x startup_seq_step_delay : Delay  DelayLength=2*startup_seq_step_delay/sample_time  UseCircularBuffer=on  SampleTime=sample_time
  Gain : Gain  Gain=2
  Gain1 : Gain  Gain=3
  Gain2 : Gain  Gain=4
  Integrator : DiscreteIntegrator  ExternalReset=either  InitialConditionSetting=State (most efficient)  SampleTime=sample_time  OutDataTypeStr=double  SaturateOnIntegerOverflow=on  LimitOutput=on  UpperSaturationLimit=6*startup_seq_step_delay  LowerSaturationLimit=0  ICPrevOutput=DiscIntNeverNeededParam  ICPrevScaledInput=DiscIntNeverNeededParam
  and5 : Logic  AllPortsSameDT=off  OutDataTypeStr=boolean
  relop{,1..3} (4 alike) : RelationalOperator  OutDataTypeStr=boolean
  startup_seq _step_delay : Constant  Value=startup_seq_step_delay  SampleTime=sample_time
  delayed : Outport
  delayed 2x : Outport  Port=2
  delayed 3x : Outport  Port=3
  delayed 4x & BR : Outport  Port=4
  (d4x & BR) delayed 2x : Outport  Port=5
  wires:
  Integrator/1 -> relop3/1, relop2/1, relop1/1, relop/1
  relop/1 -> delayed/1
  sigin/1 -> 2dbl/1
  startup_seq _step_delay/1 -> relop/2, Gain/1, Gain2/1, Gain1/1
  2dbl/1 -> Integrator/2, Integrator/1
  Gain/1 -> relop1/2
  relop1/1 -> delayed 2x/1
  Gain1/1 -> relop2/2
  relop2/1 -> delayed 3x/1
  Gain2/1 -> relop3/2
  relop3/1 -> and5/1
  2x startup_seq_step_delay/1 -> (d4x & BR) delayed 2x/1
  bus ready/1 -> and5/2
  and5/1 -> 2x startup_seq_step_delay/1, delayed 4x & BR/1

== system BugE_v0_40_MAS/Master Controller/Operating Mode Controller/Startup sequence (State 1)/zeros ==
  I : Inport
  Bus Creator : BusCreator  Inputs=5
  Bus Selector : BusSelector  OutputSignals=MB_on,SB_on,FE_on,CHG_on,LD_on
  Gain{1..5} (5 alike) : Gain  Gain=0
  bool2dbl{1..5} (5 alike) : DataTypeConversion  OutDataTypeStr=double
  dbl2bool{1..5} (5 alike) : DataTypeConversion  OutDataTypeStr=boolean
  O : Outport
  wires:
  dbl2bool1/1 -> Bus Creator/2  "SB_droop_EN"
  dbl2bool5/1 -> Bus Creator/5  "LD_droop_EN"
  I/1 -> Bus Selector/1
  dbl2bool3/1 -> Bus Creator/3  "FE_droop_EN"
  dbl2bool4/1 -> Bus Creator/4  "CHG_droop_EN"
  Bus Creator/1 -> O/1
  dbl2bool2/1 -> Bus Creator/1  "MB_droop_EN"
  bool2dbl2/1 -> Gain2/1
  Gain2/1 -> dbl2bool2/1
  Bus Selector/1 -> bool2dbl2/1  "<MB_on>"
  bool2dbl1/1 -> Gain1/1
  Gain1/1 -> dbl2bool1/1
  Bus Selector/2 -> bool2dbl1/1  "<SB_on>"
  bool2dbl3/1 -> Gain3/1
  Gain3/1 -> dbl2bool3/1
  Bus Selector/3 -> bool2dbl3/1  "<FE_on>"
  bool2dbl4/1 -> Gain4/1
  Gain4/1 -> dbl2bool4/1
  Bus Selector/4 -> bool2dbl4/1  "<CHG_on>"
  bool2dbl5/1 -> Gain5/1
  Gain5/1 -> dbl2bool5/1
  Bus Selector/5 -> bool2dbl5/1  "<LD_on>"

== system BugE_v0_40_MAS/Master Controller/Operating Mode Controller/State machine 0 std, 1 startup, 2 acc, 3 drv, 4 fault/0 => 1 ==
  Action Port : ActionPort  ActionType=elseif
  Constant : Constant
  new : Outport  InitialOutput=1
  wires:
  Constant/1 -> new/1

== system BugE_v0_40_MAS/Master Controller/Operating Mode Controller/State machine 0 std, 1 startup, 2 acc, 3 drv, 4 fault/1 => 2 ==
  Action Port : ActionPort  ActionType=elseif
  Constant : Constant  Value=2
  new : Outport  InitialOutput=1
  wires:
  Constant/1 -> new/1

== system BugE_v0_40_MAS/Master Controller/Operating Mode Controller/State machine 0 std, 1 startup, 2 acc, 3 drv, 4 fault/2 => 3 ==
  Action Port : ActionPort  ActionType=elseif
  Constant : Constant  Value=3
  new : Outport  InitialOutput=1
  wires:
  Constant/1 -> new/1

== system BugE_v0_40_MAS/Master Controller/Operating Mode Controller/State machine 0 std, 1 startup, 2 acc, 3 drv, 4 fault/3 => 2 ==
  Action Port : ActionPort  ActionType=elseif
  Constant : Constant  Value=2
  new : Outport  InitialOutput=1
  wires:
  Constant/1 -> new/1

== system BugE_v0_40_MAS/Master Controller/Operating Mode Controller/State machine 0 std, 1 startup, 2 acc, 3 drv, 4 fault/All => 0 ==
  Action Port : ActionPort  ActionType=then
  Constant : Constant  Value=0
  new : Outport  InitialOutput=1
  wires:
  Constant/1 -> new/1

== system BugE_v0_40_MAS/Master Controller/Operating Mode Controller/State machine 0 std, 1 startup, 2 acc, 3 drv, 4 fault/maintain ==
  prev : Inport
  Action Port : ActionPort  ActionType=else
  new : Outport  InitialOutput=1
  wires:
  prev/1 -> new/1
